simulink library "SUB_L4_Task_10ms_SUB_APTC"  (R2018a)
settings: Solver=VariableStepAuto  StartTime=0.0  StopTime=10.0  RelTol=1e-3
values from neighbouring files (symbols this model uses):
  APTC_TRQ_PED_TRQ_DATA_MPV = ptc_matlab_lib.PTC_MBDS_Parameter('Value', [0, 0, 0, 0, 0, 0, 0, 0, 0, 0, 0, 0, 0, 0, 0, 0 ... (first row only)    [SUB_ECU_L4_MABX_CAL.m]
  APTC_TRQ_PED_TRQ_ESPD_STEP_MPV = ptc_matlab_lib.PTC_MBDS_Parameter('Value', [500, 650, 885, 950, 1050, 1120, 1240, 1360, 1475, 1590, 1710, 1830, 1950, 2150, 2300, 2350],  	'Description', 'Pedal torque determination based on torque pedal control: input = engine speed.',  	'Unit', 'rpm')    [SUB_ECU_L4_MABX_CAL.m]
  APTC_TRQ_PED_TRQ_POS_STEP_MPV = ptc_matlab_lib.PTC_MBDS_Parameter('Value', [0, 7, 14, 21, 28, 35, 55, 100],  	'Description', 'Pedal torque determination based on torque pedal control: input = accelerator pedal position.',  	'Unit', '    [SUB_ECU_L4_MABX_CAL.m]
undefined symbols (not defined in the file or in its folder): ENUM_PEDAL_POS_SIGNAL_SOURCE_T
libraries: EmE_MBD_Blockset x6, PTC_MBDS_LIB x2
settings Model: Creator=Chris.Balton  LastModifiedBy=Gavin.Coelho

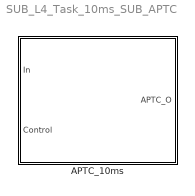
== system SUB_L4_Task_10ms_SUB_APTC ==
  APTC_10ms : Subsystem

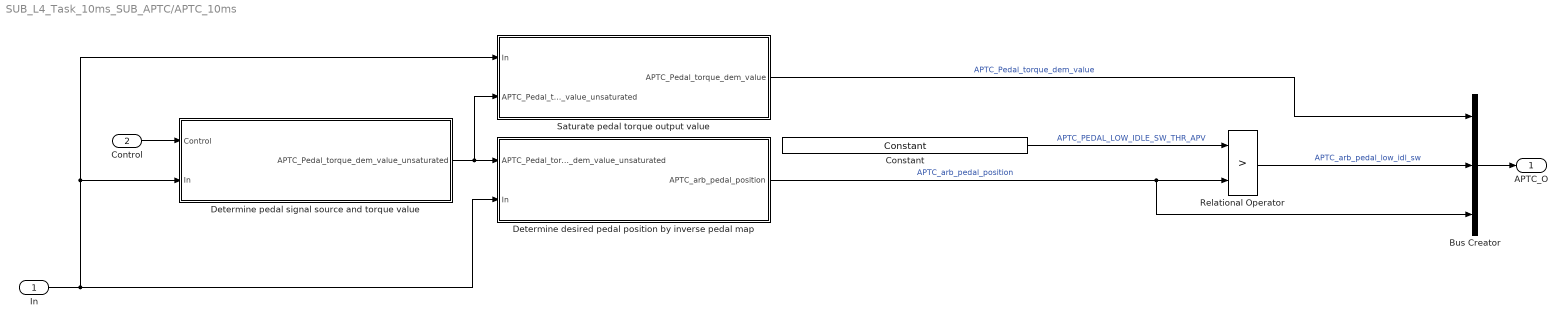
== system SUB_L4_Task_10ms_SUB_APTC/APTC_10ms ==
  In : Inport
  Control : Inport  Port=2
  Bus Creator : BusCreator  Inputs=3
  Constant : PTC_MBDS_LIB/Extras/Sources/Constant  Value2=APTC_PEDAL_LOW_IDLE_SW_THR_APV  PTC_MBDS_BlockVersion=5.41  PTC_BlockType=PTC_MBDS_Constant
      settings: SourceProductName=PACCAR Technical Center MBDS Library
      settings: AttributesFormatString=|
      | Value: 3
      | Unit: '%'
  Determine desired pedal position by inverse pedal map : Subsystem
  Determine pedal signal source and torque value : Subsystem
  Relational Operator : RelationalOperator  Operator=>  OutDataTypeStr=boolean  RndMeth=Nearest  InputSameDT=on
  Saturate pedal torque output value : Subsystem
  APTC_O : Outport
  wires:
  Determine desired pedal position by inverse pedal map/1(APTC_arb_pedal_position) -> Bus Creator/3, Relational Operator/2  "APTC_arb_pedal_position"
  Relational Operator/1 -> Bus Creator/2  "APTC_arb_pedal_low_idl_sw"
  Bus Creator/1 -> APTC_O/1
  Constant/1 -> Relational Operator/1  "APTC_PEDAL_LOW_IDLE_SW_THR_APV"
  Determine pedal signal source and torque value/1(APTC_Pedal_torque_dem_value_unsaturated) -> Determine desired pedal position by inverse pedal map/1(APTC_Pedal_torque_dem_value_unsaturated), Saturate pedal torque output value/2(APTC_Pedal_torque_dem_value_unsaturated)
  Control/1 -> Determine pedal signal source and torque value/1(Control)
  In/1 -> Saturate pedal torque output value/1(In), Determine pedal signal source and torque value/2(In), Determine desired pedal position by inverse pedal map/2(In)
  Saturate pedal torque output value/1(APTC_Pedal_torque_dem_value) -> Bus Creator/1  "APTC_Pedal_torque_dem_value"

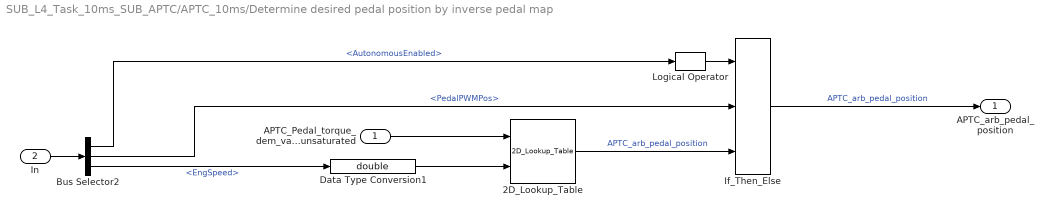
== system SUB_L4_Task_10ms_SUB_APTC/APTC_10ms/Determine desired pedal position by inverse pedal map ==
  APTC_Pedal_torque_dem_value_unsaturated : Inport
  In : Inport  Port=2
  2D_Lookup_Table : PTC_MBDS_LIB/Extras/Lookup Tables/2D_Lookup_Table  ParameterObjectName=APTC_TRQ_PED_INV_MAP_PED_POS_MPV  InterpolationMethod=Linear  PTC_MBDS_BlockVersion=5.41  PTC_BlockType=PTC_MBDS_2D_Lookup_Table
      settings: SourceProductName=PACCAR Technical Center MBDS Library
      settings: AttributesFormatString=|
      | Row Axis: APTC_TRQ_PED_INV_MAP_TRQ_STEPS (N*m)
      | Column Axis: APTC_TRQ_PED_TRQ_ESPD_STEP_MPV (rpm)
      | Data Axis: APTC_TRQ_PED_INV_MAP_PED_POS_MPV (N*m)
      | Interpolation Method: Linear
  Bus Selector2 : BusSelector  OutputSignals=AutonomousState.AutonomousEnabled,DIO_Bus.PedalPWMPos,CAN.EEC1_00.EngSpeed
  Data Type Conversion1 : DataTypeConversion  OutDataTypeStr=double
  If_Then_Else : EmE_MBD_Blockset/Signal Routing/If_Then_Else
      settings: SourceProductName=PACCAR EmE MBD Blockset
  Logical Operator : EmE_MBD_Blockset/Logic and Bit Operations/Logical Operator  Operator=NOT  Inputs=2
      settings: SourceProductName=PACCAR EmE MBD Blockset
  APTC_arb_pedal_position : Outport
  wires:
  Bus Selector2/2 -> If_Then_Else/2  "<PedalPWMPos>"
  Logical Operator/1 -> If_Then_Else/1
  Data Type Conversion1/1 -> 2D_Lookup_Table/2
  2D_Lookup_Table/1 -> If_Then_Else/3  "APTC_arb_pedal_position"
  Bus Selector2/1 -> Logical Operator/1  "<AutonomousEnabled>"
  If_Then_Else/1 -> APTC_arb_pedal_position/1  "APTC_arb_pedal_position"
  APTC_Pedal_torque_dem_value_unsaturated/1 -> 2D_Lookup_Table/1
  In/1 -> Bus Selector2/1
  Bus Selector2/3 -> Data Type Conversion1/1  "<EngSpeed>"

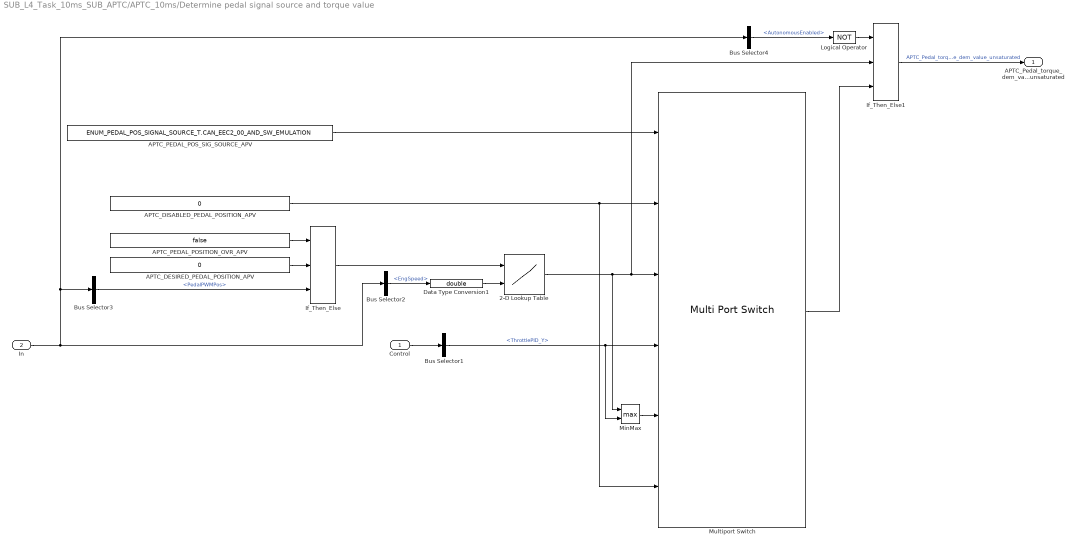
== system SUB_L4_Task_10ms_SUB_APTC/APTC_10ms/Determine pedal signal source and torque value ==
  Control : Inport
  In : Inport  Port=2
  2-D Lookup Table : Lookup_n-D  BreakpointsForDimension1=APTC_TRQ_PED_TRQ_POS_STEP_MPV  BreakpointsForDimension2=APTC_TRQ_PED_TRQ_ESPD_STEP_MPV  Table=APTC_TRQ_PED_TRQ_DATA_MPV  ExtrapMethod=Clip  UseLastTableValue=on  InputSameDT=on
      settings: AttributesFormatString=|
      | X: %<BreakpointsForDimension1>
      | Y: %<BreakpointsForDimension2>
      | Z: %<Table>
  APTC_DESIRED_PEDAL_POSITION_APV : Constant  Value=0
  APTC_DISABLED_PEDAL_POSITION_APV : Constant  Value=0
  APTC_PEDAL_POSITION_OVR_APV : Constant  Value=false
  APTC_PEDAL_POS_SIG_SOURCE_APV : Constant  Value=ENUM_PEDAL_POS_SIGNAL_SOURCE_T.CAN_EEC2_00_AND_SW_EMULATION
  Bus Selector1 : BusSelector  OutputSignals=ThrottlePID_Y
  Bus Selector2 : BusSelector  OutputSignals=CAN.EEC1_00.EngSpeed
  Bus Selector3 : BusSelector  OutputSignals=DIO_Bus.PedalPWMPos
  Bus Selector4 : BusSelector  OutputSignals=AutonomousState.AutonomousEnabled
  Data Type Conversion1 : DataTypeConversion  OutDataTypeStr=double
  If_Then_Else : EmE_MBD_Blockset/Signal Routing/If_Then_Else
      settings: SourceProductName=PACCAR EmE MBD Blockset
  If_Then_Else1 : EmE_MBD_Blockset/Signal Routing/If_Then_Else
      settings: SourceProductName=PACCAR EmE MBD Blockset
  Logical Operator : Logic  Operator=NOT  OutDataTypeStr=boolean
  MinMax : MinMax  Function=max  Inputs=2  InputSameDT=on
  Multiport Switch : MultiPortSwitch  DataPortOrder=Specify indices  Inputs={ENUM_PEDAL_POS_SIGNAL_SOURCE_T.CAN_EEC2_00, ENUM_PEDAL_POS_SIGNAL_SOURCE_T.SW_EMULATION}  DataPortIndices={ENUM_PEDAL_POS_SIGNAL_SOURCE_T.DISABLED,ENUM_PEDAL_POS_SIGNAL_SOURCE_T.CAN_EEC2_00, ENUM_PEDAL_POS_SIGNAL_SOURCE_T.SW_EMULATION,ENUM_PEDAL_POS_SIGNAL_SOURCE_T.CAN_EEC2_00_AND_SW_EMULATION}  DataPortForDefault=Additional data port  DiagnosticForDefault=None
  APTC_Pedal_torque_dem_value_unsaturated : Outport
  wires:
  Multiport Switch/1 -> If_Then_Else1/3
  Logical Operator/1 -> If_Then_Else1/1
  Bus Selector4/1 -> Logical Operator/1  "<AutonomousEnabled>"
  If_Then_Else/1 -> 2-D Lookup Table/1
  APTC_PEDAL_POSITION_OVR_APV/1 -> If_Then_Else/1
  APTC_DESIRED_PEDAL_POSITION_APV/1 -> If_Then_Else/2
  Bus Selector1/1 -> MinMax/2, Multiport Switch/4  "<ThrottlePID_Y>"
  Control/1 -> Bus Selector1/1
  If_Then_Else1/1 -> APTC_Pedal_torque_dem_value_unsaturated/1  "APTC_Pedal_torque_dem_value_unsaturated"
  2-D Lookup Table/1 -> Multiport Switch/3, If_Then_Else1/2, MinMax/1
  APTC_PEDAL_POS_SIG_SOURCE_APV/1 -> Multiport Switch/1
  MinMax/1 -> Multiport Switch/5
  APTC_DISABLED_PEDAL_POSITION_APV/1 -> Multiport Switch/6, Multiport Switch/2
  Bus Selector3/1 -> If_Then_Else/3  "<PedalPWMPos>"
  In/1 -> Bus Selector4/1, Bus Selector3/1, Bus Selector2/1
  Bus Selector2/1 -> Data Type Conversion1/1  "<EngSpeed>"
  Data Type Conversion1/1 -> 2-D Lookup Table/2

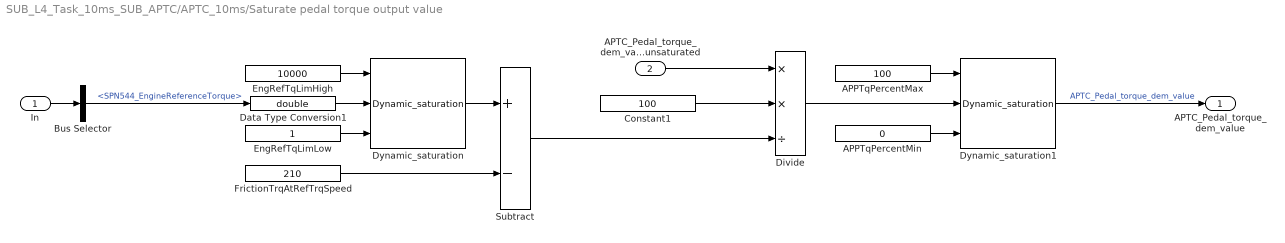
== system SUB_L4_Task_10ms_SUB_APTC/APTC_10ms/Saturate pedal torque output value ==
  In : Inport
  APTC_Pedal_torque_dem_value_unsaturated : Inport  Port=2
  APPTqPercentMax : Constant  Value=100
  APPTqPercentMin : Constant  Value=0
  Bus Selector : BusSelector  OutputSignals=CAN.EC1_00.SPN544_EngineReferenceTorque
  Constant1 : Constant  Value=100
  Data Type Conversion1 : DataTypeConversion  OutDataTypeStr=double
  Divide : Product  Inputs=**/  InputSameDT=on
  Dynamic_saturation : EmE_MBD_Blockset/Discontinuities/Dynamic_saturation
      settings: SourceProductName=PACCAR EmE MBD Blockset
  Dynamic_saturation1 : EmE_MBD_Blockset/Discontinuities/Dynamic_saturation
      settings: SourceProductName=PACCAR EmE MBD Blockset
  EngRefTqLimHigh : Constant  Value=10000
  EngRefTqLimLow : Constant
  FrictionTrqAtRefTrqSpeed : Constant  Value=210
  Subtract : Sum  Inputs=+-  InputSameDT=on
  APTC_Pedal_torque_dem_value : Outport
  wires:
  Constant1/1 -> Divide/2
  Divide/1 -> Dynamic_saturation1/2
  APPTqPercentMax/1 -> Dynamic_saturation1/1
  APPTqPercentMin/1 -> Dynamic_saturation1/3
  Subtract/1 -> Divide/3
  FrictionTrqAtRefTrqSpeed/1 -> Subtract/2
  Dynamic_saturation/1 -> Subtract/1
  EngRefTqLimHigh/1 -> Dynamic_saturation/1
  EngRefTqLimLow/1 -> Dynamic_saturation/3
  Dynamic_saturation1/1 -> APTC_Pedal_torque_dem_value/1  "APTC_Pedal_torque_dem_value"
  APTC_Pedal_torque_dem_value_unsaturated/1 -> Divide/1
  Bus Selector/1 -> Data Type Conversion1/1  "<SPN544_EngineReferenceTorque>"
  In/1 -> Bus Selector/1
  Data Type Conversion1/1 -> Dynamic_saturation/2
